simulink model "slb_trg_enable"  (R2015b)
settings: Solver=FixedStepDiscrete  SolverMode=SingleTasking  StartTime=0.0  StopTime=20  RelTol=1e-3
libraries: simulink x7
CloseFcn:
  | rtwprivate ssgencode ModelCloseRequest Hysteresis_test1
settings Model: DataTypeOverride=Off  Creator=at-mt  LastModifiedBy=amatsumo
settings DataIOCC: SaveFormat=Array  SaveOutput=off  SignalLogging=off  SaveTime=off
settings OptimizationCC: BlockReduction=off  ConditionallyExecuteInputs=off  DefaultParameterBehavior=Inlined  ExpressionDepthLimit=2147483647
settings DebuggingCC: AlgebraicLoopMsg=error  UnderspecifiedInitializationDetection=Classic  MergeDetectMultiDrivingBlocksExec=none  SolverPrmCheckMsg=warning  SingleTaskRateTransMsg=error  FcnCallInpInsideContextMsg=UseLocalSettings  StateNameClashWarn=warning
settings HardwareCC: ProdBitPerPointer=32  ProdLargestAtomicFloat=None  ProdIntDivRoundTo=Undefined  ProdEndianess=Unspecified  ProdWordSize=32  ProdHWDeviceType=ASIC/FPGA->ASIC/FPGA  ProdEqTarget=off
settings GRTTargetCC: GeneratePreprocessorConditionals=Disable all  CombineOutputUpdateFcns=off  GRTInterface=on
settings ConfigComp: CovModelRefEnable=Off  CovSFcnEnable=off

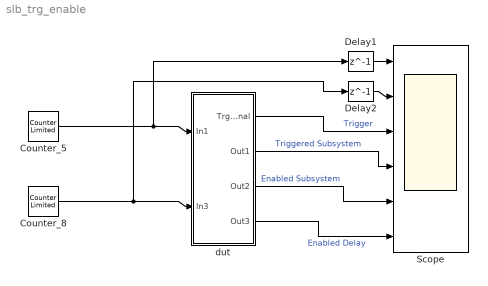
== system slb_trg_enable ==
  Counter_5 : simulink/Sources/Counter Limited  uplimit=5  tsamp=1
  Counter_8 : simulink/Sources/Counter Limited  uplimit=8  tsamp=1
  Delay1 : Delay  DelayLength=1  InputProcessing=Inherited
  Delay2 : Delay  DelayLength=1  InputProcessing=Inherited
  Scope : Scope  NumInputPorts=6
  dut : Subsystem
  wires:
  Counter_5/1 -> dut/1(In1), Delay1/1
  Counter_8/1 -> dut/2(In3), Delay2/1
  Delay1/1 -> Scope/1
  Delay2/1 -> Scope/2
  dut/1(Trg_signal) -> Scope/3  "Trigger"
  dut/2(Out1) -> Scope/4  "Triggered Subsystem"
  dut/3(Out2) -> Scope/5  "Enabled Subsystem"
  dut/4(Out3) -> Scope/6  "Enabled Delay"

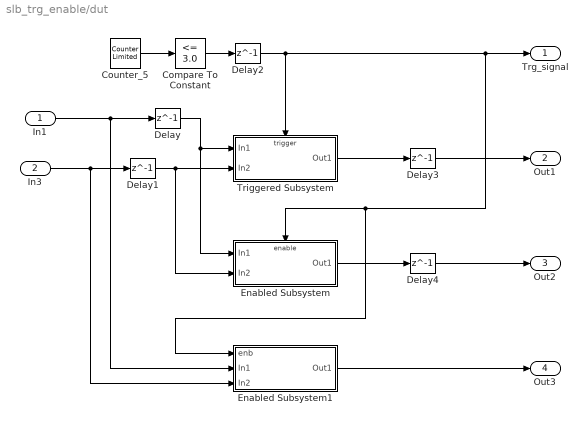
== system slb_trg_enable/dut ==
  In1 : Inport
  In3 : Inport  Port=2
  Compare To Constant : simulink/Logic and Bit Operations/Compare To Constant  relop=<=  const=3.0  OutDataTypeStr=boolean
  Counter_5 : simulink/Sources/Counter Limited  uplimit=6  tsamp=1
  Delay{,1..4} (5 alike) : Delay  DelayLength=1  InputProcessing=Inherited
  Enabled Subsystem : Subsystem  TreatAsAtomicUnit=on
  Enabled Subsystem1 : Subsystem  TreatAsAtomicUnit=on
  Triggered Subsystem : Subsystem  TreatAsAtomicUnit=on
  Trg_signal : Outport
  Out1 : Outport  Port=2
  Out2 : Outport  Port=3
  Out3 : Outport  Port=4
  wires:
  In1/1 -> Delay/1, Enabled Subsystem1/2(In1)
  In3/1 -> Delay1/1, Enabled Subsystem1/3(In2)
  Delay/1 -> Triggered Subsystem/1(In1), Enabled Subsystem/1(In1)
  Delay1/1 -> Triggered Subsystem/2(In2), Enabled Subsystem/2(In2)
  Triggered Subsystem/1(Out1) -> Delay3/1
  Enabled Subsystem/1(Out1) -> Delay4/1
  Counter_5/1 -> Compare To Constant/1
  Compare To Constant/1 -> Delay2/1
  Delay2/1 -> Triggered Subsystem/Trigger, Trg_signal/1, Enabled Subsystem/Enable, Enabled Subsystem1/1(enb)
  Delay3/1 -> Out1/1
  Delay4/1 -> Out2/1
  Enabled Subsystem1/1(Out1) -> Out3/1

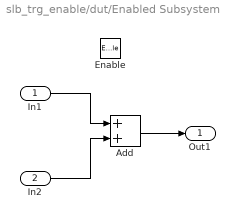
== system slb_trg_enable/dut/Enabled Subsystem ==
  In1 : Inport
  In2 : Inport  Port=2
  Enable : EnablePort
  Add : Sum
  Out1 : Outport  InitialOutput=0
  wires:
  In1/1 -> Add/1
  In2/1 -> Add/2
  Add/1 -> Out1/1

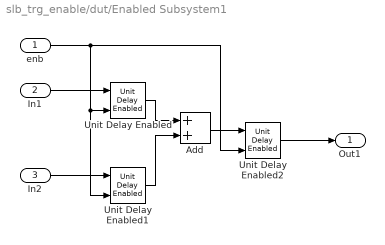
== system slb_trg_enable/dut/Enabled Subsystem1 ==
  enb : Inport
  In1 : Inport  Port=2
  In2 : Inport  Port=3
  Add : Sum
  Unit Delay Enabled : simulink/Additional Math & Discrete/Additional Discrete/Unit Delay Enabled  vinit=0.0  tsamp=-1
  Unit Delay Enabled1 : simulink/Additional Math & Discrete/Additional Discrete/Unit Delay Enabled  vinit=0.0  tsamp=-1
  Unit Delay Enabled2 : simulink/Additional Math & Discrete/Additional Discrete/Unit Delay Enabled  vinit=0.0  tsamp=-1
  Out1 : Outport  InitialOutput=0
  wires:
  In1/1 -> Unit Delay Enabled/1
  Unit Delay Enabled/1 -> Add/1
  In2/1 -> Unit Delay Enabled1/1
  Unit Delay Enabled1/1 -> Add/2
  Add/1 -> Unit Delay Enabled2/1
  Unit Delay Enabled2/1 -> Out1/1
  enb/1 -> Unit Delay Enabled/2, Unit Delay Enabled1/2, Unit Delay Enabled2/2

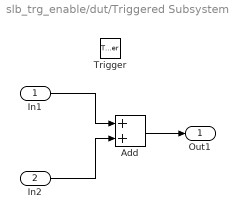
== system slb_trg_enable/dut/Triggered Subsystem ==
  In1 : Inport
  In2 : Inport  Port=2
  Trigger : TriggerPort
  Add : Sum
  Out1 : Outport  InitialOutput=0
  wires:
  In1/1 -> Add/1
  In2/1 -> Add/2
  Add/1 -> Out1/1
